simulink model "DQN_ABC_Test"  (R2023b)
settings: Solver=ode23tb  StartTime=0.0  StopTime=0.1  FixedStep=Ts  RelTol=1e-3
values from neighbouring files (symbols this model uses):
  Carm = 3.76    [DQn_ABC_Test_calc.m]
  L = Ld + Lm    [DQn_ABC_Test_calc.m]
  La = 1e-3    (= 0.001)    [DQn_ABC_Test_calc.m]
  Lb = 2*La    (= 0.002)    [DQn_ABC_Test_calc.m]
  Lc = 0.5*La    (= 0.0005)    [DQn_ABC_Test_calc.m]
  N = 1    [DQn_ABC_Test_calc.m]
  R = Rd + Rm    [DQn_ABC_Test_calc.m]
  Ra = 1.64    [DQn_ABC_Test_calc.m]
  Rb = 1.4*Ra    (= 2.296)    [DQn_ABC_Test_calc.m]
  Rc = 2.8*Ra    (= 4.592)    [DQn_ABC_Test_calc.m]
  Ta_dqn = oDP.Ta_dqn    [DQn_ABC_Test_calc.m]
  Ts = 50e-6    (= 5e-05)    [DQn_ABC_Test_calc.m]
  Ts_dqn = Ts    (= 5e-05)    [DQn_ABC_Test_calc.m]
  Ts_emt = Ts    (= 5e-05)    [DQn_ABC_Test_calc.m]
  Ws = 2*pi*f    (= 314.159265359)    [DQn_ABC_Test_calc.m]
undefined symbols (not defined in the file or in its folder): DiscIntNeverNeededParam, i, Xdcpnz, Xdcpnz_c, Xpnz, Ydcpnz, Ydcpnz_c, Ypnz
libraries: DQN_Lib x81, spsCurrentMeasurementLib x9, spsControlledVoltageSourceLib x9, spsSeriesRLCBranchLib x6, spsGroundLib x6, simulink x3, spsMutualInductanceLib x1, spspowerguiLib x1
(part 6 of 6)

== matlab function DQN_ABC_Test/ABC/Int ==
  data: x input; z output; dt parameter
function z = fcn(x, dt)

    persistent z_old;    
    persistent x_old;   
    persistent dt2;
    
    if(isempty(dt2))
        dt2 = dt/2; 
        z_old  = zeros(3,1);
        x_old  = zeros(3,1);
    end
    
    R = 1.3;
    iL = 1000;
    Krl1 = (dt2*iL/(1+dt2*R*iL));
    Krl2 = (1-dt2*R*iL)/(1+dt2*R*iL);
    
    z = zeros(3,1);

    %z = (dt2)*(x+x_old)+z_old;
    z = Krl1*(x+x_old)+Krl2*z_old;
    z_old = z;
    x_old = x;
    
end

== matlab function DQN_ABC_Test/MATLAB Function3 ==
  data: Xpnz input; Xabc output; th input; HRM parameter; X_DQN output; chkHrmLst parameter; HrmLst parameter
function [Xabc, X_DQN] = fcn(Xpnz, th, HRM, chkHrmLst, HrmLst)
abc3p = zeros(3,1);

    X_DQN = zeros((HRM+1)*6,1);
    
    if(chkHrmLst)
        range = numel(HrmLst);
    else
       range = HRM+1; 
       
    end
    
    h = 0;
    for i = 1:range
        
        if(chkHrmLst)
            h = HrmLst(i)+1;
        else
            h = i; 
        end
        
        Magp = Xpnz(1,h);
        Angp = Xpnz(2,h);
        Magn = Xpnz(3,h);
        Angn = Xpnz(4,h);
        Magz = Xpnz(5,h);
        Angz = Xpnz(6,h);

        Xdp = Magp*cos(Angp);
        Xqp = Magp*sin(Angp);
        Xdn =-Magn*cos(Angn);
        Xqn = Magn*sin(Angn);
        Xdz = Magz*cos(Angz);
        Xqz = Magz*sin(Angz);

        Tda_p = [sin((h-1)*th)            cos((h-1)*th);
                 sin((h-1)*th-2*pi/3)     cos((h-1)*th-2*pi/3);
                 sin((h-1)*th+2*pi/3)     cos((h-1)*th+2*pi/3)];

        Tda_n = [sin(-(h-1)*th)           cos(-(h-1)*th);
                 sin(-(h-1)*th-2*pi/3)    cos(-(h-1)*th-2*pi/3);
                 sin(-(h-1)*th+2*pi/3)    cos(-(h-1)*th+2*pi/3)];

        Tda_z = [sin((h-1)*th)            cos((h-1)*th);
                 sin((h-1)*th)            cos((h-1)*th);
                 sin((h-1)*th)            cos((h-1)*th)];


        Tdqn_a = [Tda_p(:,1)  Tda_n(:,1)  Tda_z(:,1)  Tda_p(:,2)  Tda_n(:,2)  Tda_z(:,2)];

        if(h==1)
            abc3p = abc3p + Tdqn_a*[Xdp;-Xdn;Xdz;Xqp;Xqn;Xqz];
            
            X_DQN(h+0*(HRM+1)) = 2*Xdp;
            X_DQN(h+1*(HRM+1)) = -2*Xdn;
            X_DQN(h+2*(HRM+1)) = 0;
            X_DQN(h+3*(HRM+1)) = 2*Xqp;
            X_DQN(h+4*(HRM+1)) = 2*Xqn;
            X_DQN(h+5*(HRM+1)) = Xqz;
            
        else
            abc3p = abc3p + Tdqn_a*[Xdp;Xdn;Xdz;Xqp;Xqn;Xqz];
            
            X_DQN(h+0*(HRM+1)) = Xdp;
            X_DQN(h+1*(HRM+1)) = Xdn;
            X_DQN(h+2*(HRM+1)) = Xdz;
            X_DQN(h+3*(HRM+1)) = Xqp;
            X_DQN(h+4*(HRM+1)) = Xqn;
            X_DQN(h+5*(HRM+1)) = Xqz;
        end
        


    end


    Xabc = abc3p;
    
end
